simulink model "PID_controller"  (R2020b)
settings: Solver=VariableStepAuto  StartTime=0.0  StopTime=15  RelTol=1e-3
values from neighbouring files (symbols this model uses):
  b = 10    [PID_Controller.m]    (also in PurePursiut_Stanley_plots.m = xRefq(ii+5) - xRefq(ii-1); Spring_Mass_Dampr.m; simulation_plots_HighwayAssist.m = xRefq(ii+5) - xRefq(ii-1); simulation_plots_week6.m = xRefq(ii+5) - xRefq(ii-1))
  k = 20    [PID_Controller.m]    (also in Spring_Mass_Dampr.m; test.m)
  kd = 25    [PID_Controller.m]
  ki = 300    [PID_Controller.m]
  kp = 350    [PID_Controller.m]
  m = 1084    [Headway_Controller_Design.m]    (also in LCA_init.m = 1140; MPC_init.m = 1140; PID_Controller.m = 1; Reduced_order_model.m)
  step_value = 1    [PID_Controller.m]    (also in Spring_Mass_Dampr.m; test.m)
settings Model: PacingRate=15  Creator=ChOm1  LastModifiedBy=ChOm1

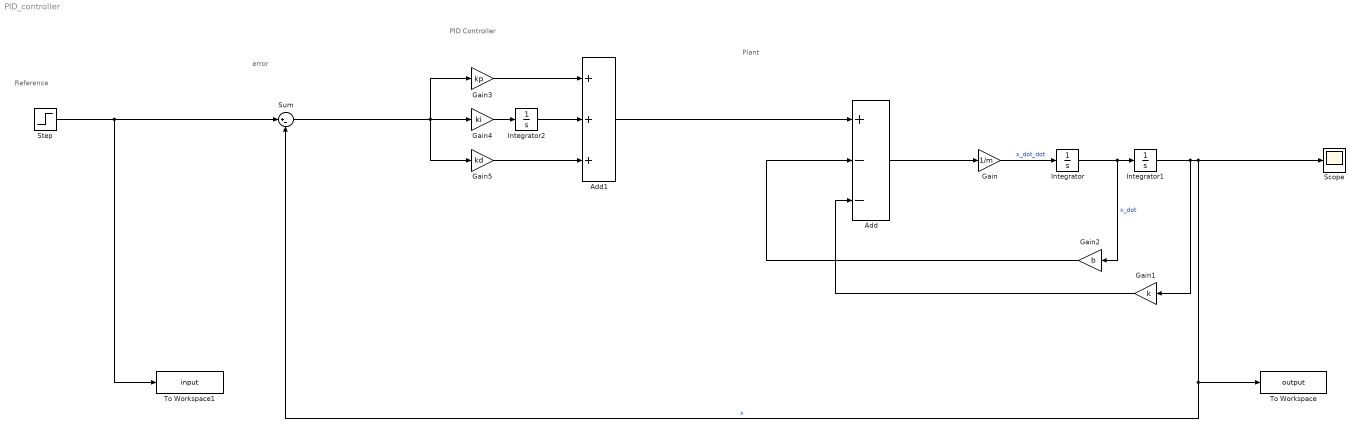
== system PID_controller ==
  note: Reference
  note: error
  note: PID Controller
  note: Plant
  Add : Sum  Inputs=+--
  Add1 : Sum  Inputs=+++
  Gain : Gain  Gain=1/m
  Gain1 : Gain  Gain=k
  Gain2 : Gain  Gain=b
  Gain3 : Gain  Gain=kp
  Gain4 : Gain  Gain=ki
  Gain5 : Gain  Gain=kd
  Integrator : Integrator
  Integrator1 : Integrator
  Integrator2 : Integrator
  Scope : Scope
  Step : Step  After=step_value  SampleTime=0
  Sum : Sum  Inputs=|+-
  To Workspace : ToWorkspace  VariableName=output  SaveFormat=Timeseries  SampleTime=-1
  To Workspace1 : ToWorkspace  VariableName=input  SaveFormat=Timeseries  SampleTime=-1
  wires:
  Add/1 -> Gain/1
  Gain/1 -> Integrator/1  "x_dot_dot"
  Integrator/1 -> Gain2/1, Integrator1/1  "x_dot"
  Integrator1/1 -> To Workspace/1, Sum/2, Scope/1, Gain1/1  "x"
  Gain2/1 -> Add/2
  Gain1/1 -> Add/3
  Gain4/1 -> Integrator2/1
  Integrator2/1 -> Add1/2
  Gain3/1 -> Add1/1
  Gain5/1 -> Add1/3
  Add1/1 -> Add/1
  Step/1 -> To Workspace1/1, Sum/1
  Sum/1 -> Gain5/1, Gain3/1, Gain4/1
